simulink model "Traffic_123"  (R2019a)
settings: Solver=VariableStepAuto  StartTime=0.0  StopTime=100  RelTol=1e-3
settings Model: Creator=HP  LastModifiedBy=HP

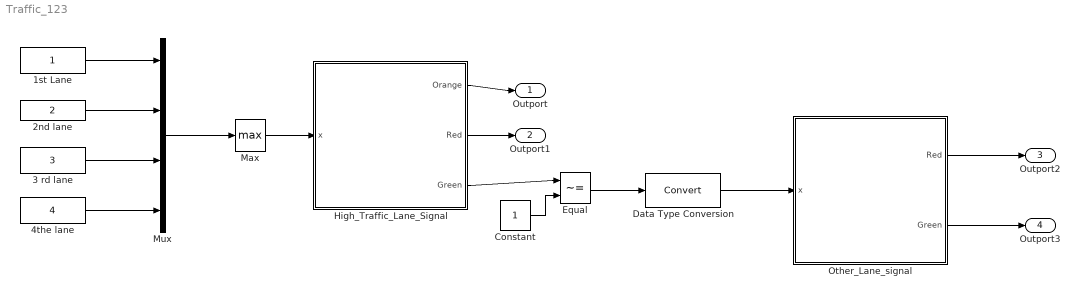
== system Traffic_123 ==
  1st Lane : Constant
  2nd lane : Constant  Value=2
  3 rd lane : Constant  Value=3
  4the lane : Constant  Value=4
  Constant : Constant
  Data Type Conversion : DataTypeConversion
  Equal : RelationalOperator  Operator=~=  OutDataTypeStr=boolean  RndMeth=Simplest
  High_Traffic_Lane_Signal : Stateflow chart  TreatAsAtomicUnit=on
  Max : MinMax  Function=max
  Mux : Mux
  Other_Lane_signal : Stateflow chart  TreatAsAtomicUnit=on
  Outport : Outport
  Outport1 : Outport  Port=2
  Outport2 : Outport  Port=3
  Outport3 : Outport  Port=4
  wires:
  1st Lane/1 -> Mux/1
  2nd lane/1 -> Mux/2
  3 rd lane/1 -> Mux/3
  4the lane/1 -> Mux/4
  Mux/1 -> Max/1
  Max/1 -> High_Traffic_Lane_Signal/1(x)
  High_Traffic_Lane_Signal/1(Orange) -> Outport/1
  High_Traffic_Lane_Signal/2(Red) -> Outport1/1
  High_Traffic_Lane_Signal/3(Green) -> Equal/1
  Constant/1 -> Equal/2
  Equal/1 -> Data Type Conversion/1
  Data Type Conversion/1 -> Other_Lane_signal/1(x)
  Other_Lane_signal/1(Red) -> Outport2/1
  Other_Lane_signal/2(Green) -> Outport3/1

== stateflow chart Traffic_123/Other_Lane_signal ==
  state Stop
    Red=0;
    Green=1;
  state Start
    Red=1;
    Green=0;
  (default) -> Start
  Start -> Stop : after(60,sec)
  data: x input; Red output; Green output; Orange local

== stateflow chart Traffic_123/High_Traffic_Lane_Signal ==
  state a_st
    Red=0;
    Green=0;
    Orange=1;
  state a_st1
    Red=1;
    Green=0;
    Orange=0;
  state Start
    Red=0;
    Green=1;
    Orange=0;
  (default) -> Start
  a_st -> a_st1 : after(10,sec)
  Start -> a_st : after(60,sec)
  data: x input; Orange output; Red output; Green output
